simulink model "observador_multirate_4"  (R2012b)
settings: Solver=ode3  StartTime=0.0  StopTime=20  FixedStep=1e-4  MaxStep=1e-4  RelTol=1e-3
values from neighbouring files (symbols this model uses):
  A = [-0.2  0; 1  0]    [teste_AxBu_AxBuLy_cadaumcomsuataxaindividual.mat]    (also in testes2.mat)
  B = [10 0]    [teste_AxBu_AxBuLy_cadaumcomsuataxaindividual.mat]    (also in testes2.mat)
  C = [0 1]    [teste_AxBu_AxBuLy_cadaumcomsuataxaindividual.mat]    (also in testes2.mat)
libraries: simulink x3, Encoder x1
settings Model: Creator=Juliano  LastModifiedBy=Juliano
settings DataIOCC: LimitDataPoints=off

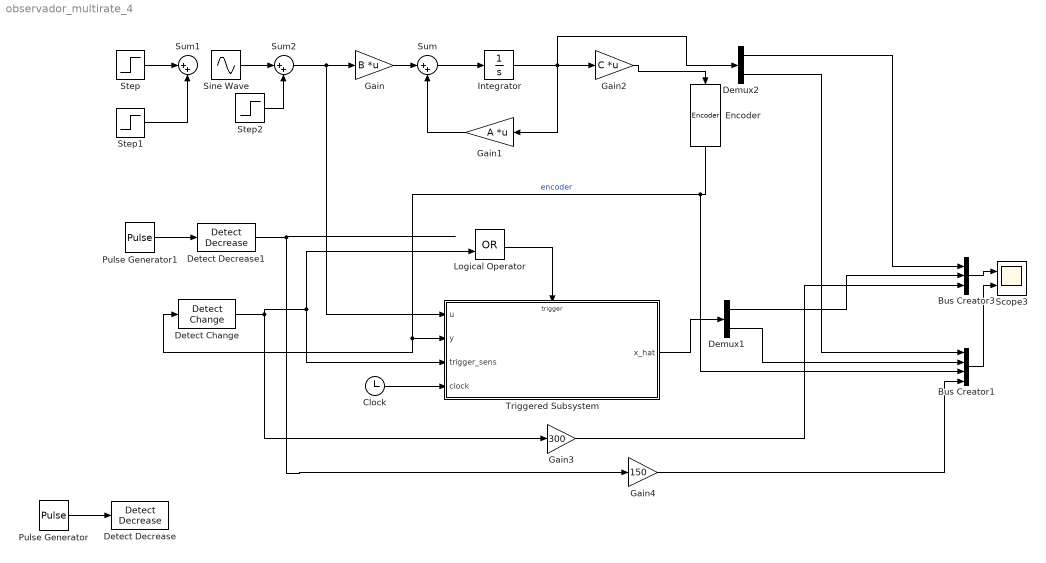
== system observador_multirate_4 ==
  Bus Creator1 : BusCreator
  Bus Creator3 : BusCreator  Inputs=3
  Clock : Clock
  Demux1 : Demux  Outputs=2
  Demux2 : Demux  Outputs=2
  Detect Change : simulink/Logic and Bit Operations/Detect Change  vinit=0  InputProcessing=Inherited  OutDataTypeStr=boolean
  Detect Decrease : simulink/Logic and Bit Operations/Detect Decrease  vinit=0.0  InputProcessing=Inherited  OutDataTypeStr=boolean
  Detect Decrease1 : simulink/Logic and Bit Operations/Detect Decrease  vinit=0.0  InputProcessing=Inherited  OutDataTypeStr=boolean
  Encoder : Encoder/Encoder  Nr=3
  Gain : Gain  Gain=B  Multiplication=Matrix(K*u)
  Gain1 : Gain  Gain=A  Multiplication=Matrix(K*u)
  Gain2 : Gain  Gain=C  Multiplication=Matrix(K*u)
  Gain3 : Gain  Gain=300  OutDataTypeStr=double
  Gain4 : Gain  Gain=150  OutDataTypeStr=double
  Integrator : Integrator
  Logical Operator : Logic  Operator=OR  AllPortsSameDT=off  OutDataTypeStr=boolean
  Pulse Generator : DiscretePulseGenerator  PulseType=Time based  Period=0.5  PulseWidth=50
  Pulse Generator1 : DiscretePulseGenerator  PulseType=Time based  Period=0.05  PulseWidth=50
  Scope3 : Scope  NumInputPorts=2
      settings: ShowLegends=on  TimeRange=10  YMin=-35000~-5  YMax=50000~5  SaveName=ScopeData2
  Sine Wave : Sin  Amplitude=20  Frequency=0.5  SampleTime=0
  Step : Step  Time=0  After=20  SampleTime=0
  Step1 : Step  Time=5  After=-40  SampleTime=0
  Step2 : Step  Time=0  After=7  SampleTime=0
  Sum : Sum  Inputs=|++
  Sum1 : Sum  Inputs=|++
  Sum2 : Sum  Inputs=|++
  Triggered Subsystem : Subsystem  TreatAsAtomicUnit=on
  wires:
  Gain/1 -> Sum/1
  Gain1/1 -> Sum/2
  Sum/1 -> Integrator/1
  Integrator/1 -> Demux2/1, Gain2/1, Gain1/1
  Step/1 -> Sum1/1
  Step1/1 -> Sum1/2
  Gain2/1 -> Encoder/1
  Bus Creator3/1 -> Scope3/1
  Pulse Generator1/1 -> Detect Decrease1/1
  Sum2/1 -> Triggered Subsystem/1(u), Gain/1
  Logical Operator/1 -> Triggered Subsystem/Trigger
  Detect Decrease1/1 -> Gain4/1
  Detect Change/1 -> Logical Operator/2, Triggered Subsystem/3(trigger_sens), Gain3/1
  Triggered Subsystem/1(x_hat) -> Demux1/1
  Demux1/1 -> Bus Creator3/2
  Pulse Generator/1 -> Detect Decrease/1
  Gain3/1 -> Bus Creator3/3
  Demux1/2 -> Bus Creator1/2
  Bus Creator1/1 -> Scope3/2
  Gain4/1 -> Bus Creator1/4
  Clock/1 -> Triggered Subsystem/4(clock)
  Encoder/1 -> Bus Creator1/3, Detect Change/1, Triggered Subsystem/2(y)  "encoder"
  Demux2/2 -> Bus Creator1/1
  Demux2/1 -> Bus Creator3/1
  Sine Wave/1 -> Sum2/1
  Step2/1 -> Sum2/2

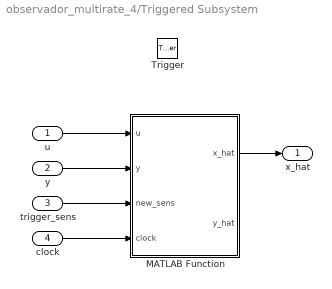
== system observador_multirate_4/Triggered Subsystem ==
  u : Inport
  y : Inport  Port=2
  trigger_sens : Inport  Port=3
  clock : Inport  Port=4
  Trigger : TriggerPort
  MATLAB Function : MATLAB Function  TreatAsAtomicUnit=on
  x_hat : Outport
  wires:
  MATLAB Function/1(x_hat) -> x_hat/1
  u/1 -> MATLAB Function/1(u)
  y/1 -> MATLAB Function/2(y)
  trigger_sens/1 -> MATLAB Function/3(new_sens)
  clock/1 -> MATLAB Function/4(clock)

== matlab function observador_multirate_4/Triggered Subsystem/MATLAB Function ==
  data: u input; y input; new_sens input; x_hat output; clock input; y_hat output
function [x_hat,y_hat] = fcn(u, y, new_sens, clock)

    %#codegen
    persistent x;
    persistent x_sens;
    persistent t;
    persistent t_sens;
    persistent C;
    persistent D;

    if(isempty(x))
        x = [0 ; 0];
        x_sens = x;
        t = -0.1;
        t_sens = t;
        C = [0 1];
        D = 0;
    end

     if(new_sens == 1)
        deltaT = clock-t_sens;
        A = [1-0.2*deltaT 0 ; deltaT 1];
        B = [10*deltaT; 0];
        L = [-0.18+0.2/deltaT+0.04*deltaT; 0.9-0.2*deltaT];
        x = A*x_sens+B*u+L*(y-C*x_sens);
        t_sens = clock;
        x_sens = x;
     else
        deltaT = clock-max(t,t_sens);
        A = [1-0.2*deltaT 0 ; deltaT 1];
        B = [10*deltaT; 0];
        x = A*x+B*u;
        t = clock;
    end
    
    x_hat = x;
    y_hat = C*x+D*u;
end
